simulink model "smarthome"  (R2024a)
settings: Solver=VariableStepAuto  StartTime=0.0  StopTime=3600  RelTol=1e-3
values from neighbouring files (symbols this model uses):
  Ag = 1.2*1.2    (= 1.44)    [home.m]
  c = 1005    [home.m]
  Fc = 0.9    [home.m]
  M = 60    [home.m]
  Mdot = 0.166    [home.m]
  Qsg = 200    [home.m]
  Req = 0.005371136080    (= 0.00537113608)    [home.m]
  THeater = 25    [home.m]
  TinIC = 9    [home.m]
  Ug = 0.35    [home.m]
libraries: fl_lib x4, nesl_utility x3, fuzblock x2, slpidlib x1
settings Model: Creator=ameer  LastModifiedBy=yadhu

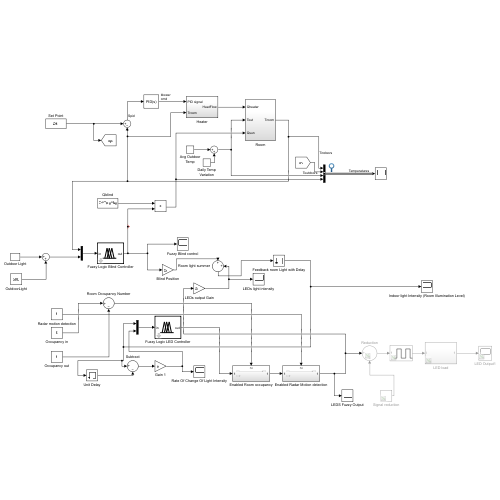
[thumbnail: Simulink's stored preview of the top-level diagram]
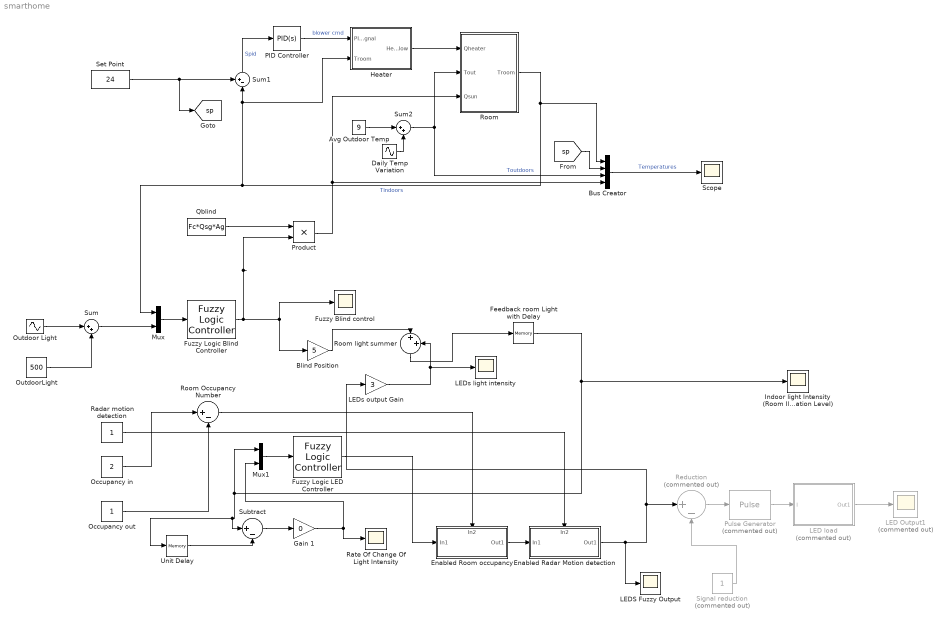
== system smarthome ==
  Avg Outdoor Temp : Constant  Value=9
  Blind Position : Gain  Gain=5
  Bus Creator : BusCreator  Inputs=4
  Daily Temp Variation : Sin  Amplitude=10  Frequency=(2*pi)/(24*3600)  SampleTime=0
  Enabled Radar Motion detection : Subsystem
      settings: PortSchema="{\"entries\":[{\"content\":{\"sides\":[{\"content\":{\"connectorIds\":[\"In1\"]},\"type\":\"ConnectorPlacement.EquallySpacedRectSide\",\"uuid\":\"51cb038c-3520-4cba-8603-e4f437bba576\"},{\"content\":{\"connectorIds\":[\"Out1\"],\"side\":\"RIGHT\"},\"type\":\"ConnectorPlacement.EquallySpacedRectSide\",\"uuid\":\"ac40f817-fdd5-427e-97bc-71021c235469\"},{\"content\":{\"connectorIds\":[\"In2\"],\"side\":\"TOP\"},\"type\":\"ConnectorPlacement.EquallySpacedRectSide\",\"uuid\":\"7e90b56d-87d4-4daa-8b51-d1c871182f22\"}]},\"type\":\"ConnectorPlacement.EquallySpacedConnector\",\"uuid\":\"0cc98bf1-bafa-412d-93af-b8cb2c9b29b7\"}],\"packageUris\":[\"http://schema.mathworks.com/mf0/Connector/R2020b\"],\"version\":\"1.0\"}"
  Enabled Room occupancy : Subsystem
      settings: PortSchema="{\"entries\":[{\"content\":{\"sides\":[{\"content\":{\"connectorIds\":[\"In1\"]},\"type\":\"ConnectorPlacement.EquallySpacedRectSide\",\"uuid\":\"51cb038c-3520-4cba-8603-e4f437bba576\"},{\"content\":{\"connectorIds\":[\"Out1\"],\"side\":\"RIGHT\"},\"type\":\"ConnectorPlacement.EquallySpacedRectSide\",\"uuid\":\"ac40f817-fdd5-427e-97bc-71021c235469\"},{\"content\":{\"connectorIds\":[\"In2\"],\"side\":\"TOP\"},\"type\":\"ConnectorPlacement.EquallySpacedRectSide\",\"uuid\":\"7e90b56d-87d4-4daa-8b51-d1c871182f22\"}]},\"type\":\"ConnectorPlacement.EquallySpacedConnector\",\"uuid\":\"0cc98bf1-bafa-412d-93af-b8cb2c9b29b7\"}],\"packageUris\":[\"http://schema.mathworks.com/mf0/Connector/R2020b\"],\"version\":\"1.0\"}"
  Feedback room Light with Delay : Memory
  Fuzzy Blind control : Scope
  Fuzzy Logic Blind Controller : fuzblock/Fuzzy Logic  Controller  FIS=BlindControlfinal  OutputSampleNumber=101  DataType=double  FuzzifiedInputs=off  RuleFiringStrengths=off  RuleOutputs=off  AggregatedOutputs=off  SimulateUsing=Interpreted execution  OutOfRangeInputValueMessage=warning  NoRuleFiredMessage=warning  EmptyOutputFuzzySetMessage=warning
  Fuzzy Logic LED Controller : fuzblock/Fuzzy Logic  Controller  FIS=LED_Lighting_Control_FIS  OutputSampleNumber=101  DataType=double  FuzzifiedInputs=off  RuleFiringStrengths=off  RuleOutputs=off  AggregatedOutputs=off  SimulateUsing=Interpreted execution  OutOfRangeInputValueMessage=warning  NoRuleFiredMessage=warning  EmptyOutputFuzzySetMessage=warning
  Gain 1 : Gain  Gain=0
  Heater : Subsystem
  Indoor light Intensity (Room Illumination Level) : Scope
  LED Output1 : Scope  Commented=on
  LED load : Subsystem  Commented=on
  LEDS Fuzzy Output : Scope
  LEDs light intensity : Scope
  LEDs output Gain : Gain  Gain=3
  Mux : Mux  Inputs=2
  Mux1 : Mux  Inputs=2
  Occupancy in : Constant  Value=2  OutMin=[0]  OutMax=[2]
  Occupancy out : Constant  OutMin=[0]  OutMax=[2]
  Outdoor Light : Sin  Amplitude=500  Frequency=(2*pi)/(1*3600)  SampleTime=0
  OutdoorLight : Constant  Value=500  OutMin=[0]  OutMax=[1000]
  PID Controller : slpidlib/PID Controller  Controller=PID  Form=Parallel  TimeDomain=Continuous-time  UseExternalTs=off  SampleTime=-1  IntegratorMethod=Forward Euler  FilterMethod=Forward Euler  ControllerParametersSource=internal  P=1  I=0.1  UseKiTs=off  D=0.01  UseExternalDerivativeSource=off  N=100  UseFilter=on  TunerSelectOption=Transfer Function Based (PID Tuner App)  InitialConditionSource=internal  InitialConditionForIntegrator=0  InitialConditionForFilter=0  DifferentiatorICPrevScaledInput=0  ExternalReset=none  TrackingMode=off  Kt=1  LimitOutput=off  SatLimitsSource=internal  UpperSaturationLimit=inf  LowerSaturationLimit=-inf  LinearizeAsGain=on  AntiWindupMode=none  Kb=1  LimitIntegrator=off  UpperIntegratorSaturationLimit=inf  LowerIntegratorSaturationLimit=-inf  POutMin=[]  POutMax=[]  IOutMin=[]  IOutMax=[]  DOutMin=[]  DOutMax=[]  NOutMin=[]  NOutMax=[]  SumOutMin=[]  SumOutMax=[]  SaturationOutMin=[]  SaturationOutMax=[]  PParamMin=[]  PParamMax=[]  IParamMin=[]  IParamMax=[]  DParamMin=[]  DParamMax=[]  NParamMin=[]  NParamMax=[]  KbParamMin=[]  KbParamMax=[]  KtParamMin=[]  KtParamMax=[]  KbOutMin=[]  KbOutMax=[]  KtOutMin=[]  KtOutMax=[]  IntegratorOutMin=[]  IntegratorOutMax=[]  FilterOutMin=[]  FilterOutMax=[]  SumI1OutMin=[]  SumI1OutMax=[]  SumI2OutMin=[]  SumI2OutMax=[]  SumI3OutMin=[]  SumI3OutMax=[]  SumI4OutMin=[]  SumI4OutMax=[]  SumDOutMin=[]  SumDOutMax=[]  DifferentiatorOutMin=[]  DifferentiatorOutMax=[]  FilterDiffOutCoefMin=[]  FilterDiffOutCoefMax=[]  ReciprocalOutMin=[]  ReciprocalOutMax=[]  SumDenOutMin=[]  SumDenOutMax=[]  SumNumOutMin=[]  SumNumOutMax=[]  DivideOutMin=[]  DivideOutMax=[]  UdiffTsProdOutMin=[]  UdiffTsProdOutMax=[]  NTsProdOutMin=[]  NTsProdOutMax=[]  UintegralTsProdOutMin=[]  UintegralTsProdOutMax=[]  UngainTsProdOutMin=[]  UngainTsProdOutMax=[]  ClampingZeroOutDataTypeStr=Inherit: Inherit via back propagation  ClampingZeroOutMin=[]  ClampingZeroOutMax=[]  FilterDenConstantOutDataTypeStr=Inherit: Inherit via back propagation  FilterDenConstantOutMin=[]  FilterDenConstantOutMax=[]  PCopyOutDataTypeStr=Inherit: Inherit via back propagation  PCopyOutMin=[]  PCopyOutMax=[]  NCopyOutDataTypeStr=Inherit: Inherit via back propagation  NCopyOutMin=[]  NCopyOutMax=[]  IntegratorContinuousStateAttributes=''  IntegratorStateMustResolveToSignalObject=off  IntegratorRTWStateStorageClass=Auto  FilterContinuousStateAttributes=''  FilterStateMustResolveToSignalObject=off  FilterRTWStateStorageClass=Auto  ParallelPVariant=InternalParameters  IdealPVariant=Disabled  IVariant=InternalParameters  DVariant=InternalParameters  IntegratorVariant=Continuous  SatVariant=Disabled  AWVariant=Passthrough  PCopyVariant=Disabled  TRVariant=Disabled  FdbkBlocksVariant=Forward  IdealPFdbkVariant=Disabled  SatFdbkVariant=Disabled  DerivativeFilterVariant=ContFilter  NVariant=InternalParameters  NCopyVariant=Disabled  FilterICVariant=InternalICsFilter  IntegratorICVariant=InternalICs  ExternalResetVariant=Disabled  TRSumVariant=Passthrough  SumFdbkVariant=Disabled  SumVariant=Sum_PID  TsampFilterVariant=InternalTs  TsampNgainVariant=Passthrough  TsampIntegralVariant=Disabled_SignalSpec  ExternalSaturationOutDataTypeStr=Inherit: Same as second input  DerivativeSourceVariant=ErrorSignal
  Product : Product
  Pulse Generator : DiscretePulseGenerator  Commented=on  PulseType=Time based  TimeSource=Use external signal  Period=10  PulseWidth=5
  Qblind : Constant  Value=Fc*Qsg*Ag
  Radar motion detection : Constant
  Rate Of Change Of Light Intensity : Scope
  Reduction : Sum  Commented=on  Inputs=|+-
  Room : Subsystem
  Room Occupancy Number : Sum  Inputs=|+-
  Room light summer : Sum  Inputs=|++
  Scope : Scope
  Set Point : Constant  Value=24
  Signal reduction : Constant  Commented=on
  Subtract : Sum  Inputs=|+-
  Sum : Sum  Inputs=|++
  Sum1 : Sum  Inputs=+-|  InputSameDT=on  SaturateOnIntegerOverflow=on  OutDataTypeStr=Inherit: Same as first input
  Sum2 : Sum  Inputs=|++  InputSameDT=on  SaturateOnIntegerOverflow=on  OutDataTypeStr=Inherit: Same as first input
  Unit Delay : Memory
  tag scope: sp=global
  wires:
  Blind Position/1 -> Room light summer/1
  Feedback room Light with Delay/1 -> Indoor light Intensity (Room Illumination Level)/1, Mux1/1, Unit Delay/1, Subtract/1
  LEDs output Gain/1 -> Room light summer/2, LEDs light intensity/1
  Fuzzy Logic Blind Controller/1 -> Product/2, Fuzzy Blind control/1, Blind Position/1
  Room light summer/1 -> Feedback room Light with Delay/1
  Mux/1 -> Fuzzy Logic Blind Controller/1
  Mux1/1 -> Fuzzy Logic LED Controller/1
  Occupancy in/1 -> Room Occupancy Number/1
  Occupancy out/1 -> Room Occupancy Number/2
  Unit Delay/1 -> Subtract/2
  Subtract/1 -> Gain 1/1
  Gain 1/1 -> Mux1/2, Rate Of Change Of Light Intensity/1
  Signal reduction/1 -> Reduction/2
  Radar motion detection/1 -> Enabled Radar Motion detection/2(In2)
  Fuzzy Logic LED Controller/1 -> Enabled Room occupancy/1(In1)
  Room Occupancy Number/1 -> Enabled Room occupancy/2(In2)
  Enabled Room occupancy/1(Out1) -> Enabled Radar Motion detection/1(In1)
  Enabled Radar Motion detection/1(Out1) -> LEDS Fuzzy Output/1, Reduction/1, LEDs output Gain/1
  Reduction/1 -> Pulse Generator/1
  OutdoorLight/1 -> Sum/2
  Outdoor Light/1 -> Sum/1
  Product/1 -> Bus Creator/4, Room/3(Qsun)
  Heater/1(HeatFlow) -> Room/1(Qheater)
  PID Controller/1 -> Heater/1(PID signal)  "blower cmd"
  Daily Temp Variation/1 -> Sum2/2
  [sp] -> Bus Creator/2
  Avg Outdoor Temp/1 -> Sum2/1
  Sum1/1 -> PID Controller/1  "Spid"
  Set Point/1 -> Sum1/1, [sp]
  Sum2/1 -> Bus Creator/3, Room/2(Tout)  "Toutdoors"
  Bus Creator/1 -> Scope/1  "Temperatures"
  Room/1(Troom) -> Bus Creator/1, Mux/1, Heater/2(Troom), Sum1/2  "Tindoors"
  Qblind/1 -> Product/1
  Sum/1 -> Mux/2
  Pulse Generator/1 -> LED load/1(l)
  LED load/1(Out1) -> LED Output1/1

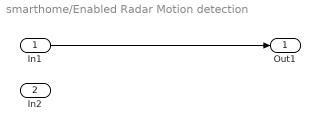
== system smarthome/Enabled Radar Motion detection ==
  In1 : Inport
  In2 : Inport  Port=2
  Out1 : Outport
  wires:
  In1/1 -> Out1/1

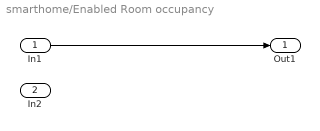
== system smarthome/Enabled Room occupancy ==
  In1 : Inport
  In2 : Inport  Port=2
  Out1 : Outport
  wires:
  In1/1 -> Out1/1

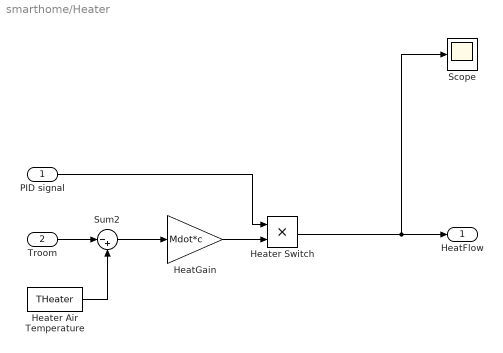
== system smarthome/Heater ==
  PID signal : Inport
  Troom : Inport  Port=2
  HeatGain : Gain  Gain=Mdot*c
  Heater Air Temperature : Constant  Value=THeater
  Heater Switch : Product  RndMeth=Zero
  Scope : Scope
  Sum2 : Sum  Inputs=|-+
  HeatFlow : Outport  VectorParamsAs1DForOutWhenUnconnected=off
  wires:
  Heater Air Temperature/1 -> Sum2/2
  Troom/1 -> Sum2/1
  Sum2/1 -> HeatGain/1
  PID signal/1 -> Heater Switch/1
  HeatGain/1 -> Heater Switch/2
  Heater Switch/1 -> Scope/1, HeatFlow/1

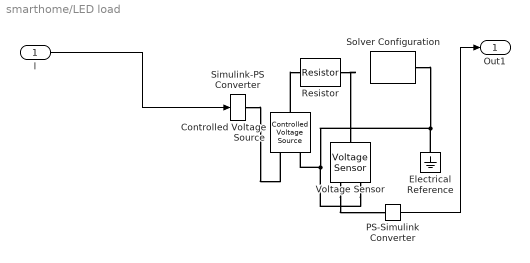
== system smarthome/LED load ==
  l : Inport
  Controlled Voltage Source : fl_lib/Electrical/Electrical Sources/Controlled Voltage Source
  Electrical Reference : fl_lib/Electrical/Electrical Elements/Electrical Reference
  PS-Simulink Converter : nesl_utility/PS-Simulink Converter  PhysicalDomain=network_engine_domain  SubClassName=ps_output  LeftPortType=input  RightPortType=output  PseudoPeriodic=off  Frequencies=[]  VectorFormat=inherit  Unit=inherit  AffineConversion=off
  Resistor : fl_lib/Electrical/Electrical Elements/Resistor  R=1 Ohm  i_specify=off  i_priority=None  i=0 A  i_nominal_specify=off  i_nominal_value=1  i_nominal_unit=A  v_specify=off  v_priority=None  v=0 V  v_nominal_specify=off  v_nominal_value=1  v_nominal_unit=V
  Simulink-PS Converter : nesl_utility/Simulink-PS Converter  PhysicalDomain=network_engine_domain  SubClassName=ps_input  LeftPortType=input  RightPortType=output  PseudoPeriodic=off  Frequencies=[]  NoiseDistribution=none  NoiseParameters=[]  Unit=1  AffineConversion=off  FilteringAndDerivatives=provide  SimscapeFilterOrder=1  InputFilterTimeConstant=0.001  UdotUserProvided=0
  Solver Configuration : nesl_utility/Solver Configuration  PhysicalDomain=network_engine_domain  SubClassName=solver  LeftPortType=input  RightPortType=generic  Tones=[]  Harmonics=[]  SimulateNoise=off  Profile=off  UseLocalSampling=off  EnableSwitchedLinearOptims=on  FrequencyDomain=off  UseCCode=off  RelTol=0.001  AbsTol=0.001  MinStep=1e-09  ToWorkspace=off  RevertToSquareIcSolve=off  NumHomotopyIterations=100  PhasorMode=off  PhasorModeNumHarmonics=1  ConsistencySolver=NEWTON_XTOL_AFTER_FTOL  IndexReductionMethod=DerivativeReplacement  DoDC=off  ResidualTolerance=1e-09  ConsistencyTolSource=GLOBAL  ConsistencyAbsTol=0.001  ConsistencyRelTol=0.001  ConsistencyTolFactor=0.001  UseLocalSolver=off  LocalSolverChoice=NE_BACKWARD_EULER_ADVANCER  ResolveIndetEquations=on  FunctionEvalNumThread=1  LocalSolverSampleTime=0.001  DoFixedCost=off  MaxNonlinIter=3  MaxModeIter=2  ComputeImpulses=off  ImpulseIterations=2  LinearAlgebra=auto  LinearAlgebraNumThread=0  EquationFormulation=NE_TIME_EF  DelaysMemoryBudget=1024  AutomaticFiltering=on  FilteringTimeConstant=0.001  PartitionStorageMethod=AS_NEEDED  PartitionMemoryBudget=1024  PartitionMethod=ROBUST  MultibodyUseLocalSolver=off  MultibodyLocalSolverChoice=ODE1  MultibodyLocalSolverSampleTime=0.001
  Voltage Sensor : fl_lib/Electrical/Electrical Sensors/Voltage Sensor
  Out1 : Outport
  wires:
  l/1 -> Simulink-PS Converter/1
  PS-Simulink Converter/1 -> Out1/1
  connections:
  Controlled Voltage Source/RConn2 -- Electrical Reference/LConn1 -- Solver Configuration/RConn1 -- Voltage Sensor/RConn2
  Resistor/RConn1 -- Voltage Sensor/LConn1
  Simulink-PS Converter/RConn1 -- Controlled Voltage Source/RConn1
  Controlled Voltage Source/LConn1 -- Resistor/LConn1
  Voltage Sensor/RConn1 -- PS-Simulink Converter/LConn1

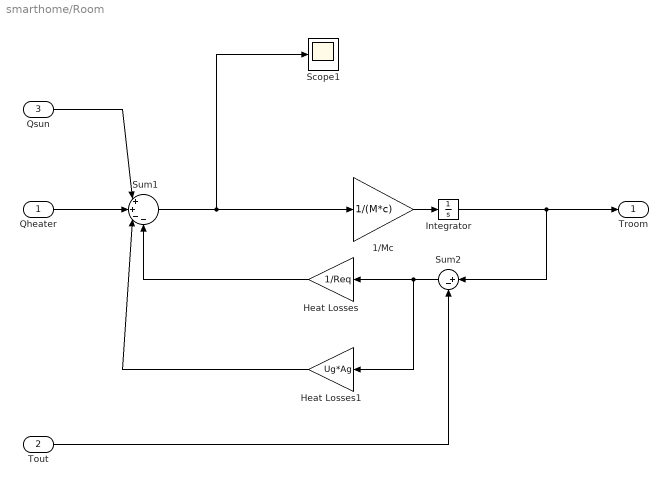
== system smarthome/Room ==
  Qheater : Inport
  Tout : Inport  Port=2
  Qsun : Inport  Port=3
  1/Mc : Gain  Gain=1/(M*c)  SaturateOnIntegerOverflow=on  OutDataTypeStr=Inherit: Same as input  ParamDataTypeStr=Inherit: Same as input
  Heat Losses : Gain  Gain=1/Req  SaturateOnIntegerOverflow=on  OutDataTypeStr=Inherit: Same as input  ParamDataTypeStr=Inherit: Same as input
  Heat Losses1 : Gain  Gain=Ug*Ag  SaturateOnIntegerOverflow=on  OutDataTypeStr=Inherit: Same as input  ParamDataTypeStr=Inherit: Same as input
  Integrator : Integrator  InitialCondition=TinIC
  Scope1 : Scope
  Sum1 : Sum  Inputs=|++--  InputSameDT=on  SaturateOnIntegerOverflow=on  OutDataTypeStr=Inherit: Same as first input
  Sum2 : Sum  Inputs=|+-  InputSameDT=on  SaturateOnIntegerOverflow=on  OutDataTypeStr=Inherit: Same as first input
  Troom : Outport  InitialOutput=0  VectorParamsAs1DForOutWhenUnconnected=off
  wires:
  Tout/1 -> Sum2/2
  Qheater/1 -> Sum1/2
  Sum1/1 -> Scope1/1, 1/Mc/1
  Sum2/1 -> Heat Losses1/1, Heat Losses/1
  1/Mc/1 -> Integrator/1
  Integrator/1 -> Troom/1, Sum2/1
  Heat Losses/1 -> Sum1/4
  Heat Losses1/1 -> Sum1/3
  Qsun/1 -> Sum1/1
